simulink library "gsWave_cl"  (R2020a)
settings: Solver=VariableStepAuto  StartTime=0.0  StopTime=10.0  RelTol=1e-3
undefined symbols (not defined in the file): gndStn
libraries: eulAng2RotMat_ul x1, simulink x1, firstOrdTrnsThm_ul x1
settings Model: Creator=M.Cobb  LastModifiedBy=adabney
settings DataIOCC: ReturnWorkspaceOutputs=off
settings DebuggingCC: ArithmeticOperatorsInVariantConditions=warning
settings SFSimCC: CustomCodeUndefinedFunction=UseInterfaceOnly

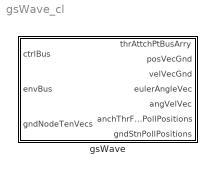
== system gsWave_cl ==
  gsWave : Subsystem  mask{gs=0}
      mask prompts: gs "Ground station object"

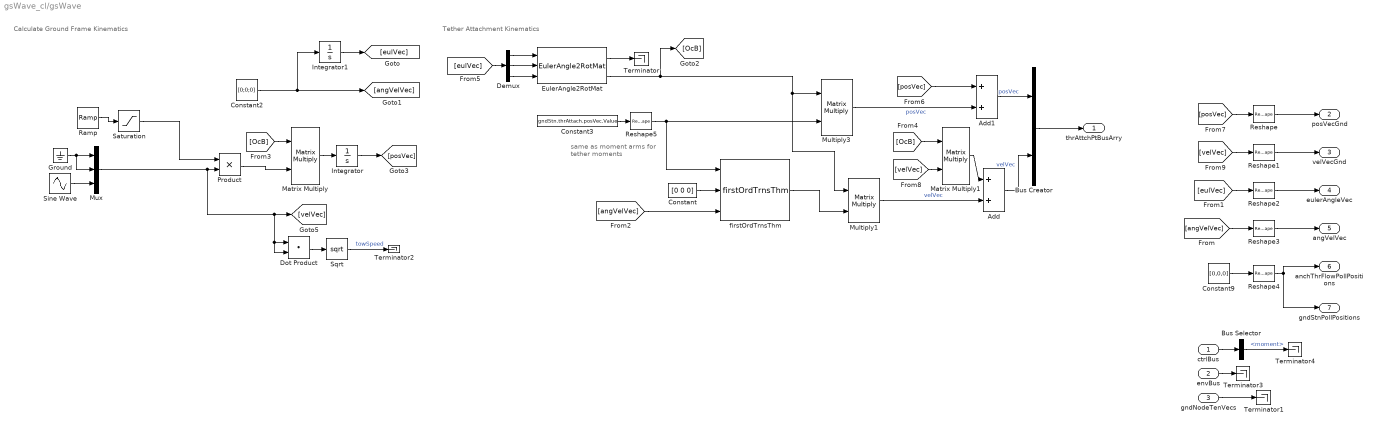
== system gsWave_cl/gsWave ==
  note: Tether Attachment Kinematics
  note: Calculate Ground Frame Kinematics
  note: same as moment arms
      | for tether moments
  ctrlBus : Inport  OutDataTypeStr=Bus: gndStnCtrlBus
  envBus : Inport  Port=2  OutDataTypeStr=Bus: envBus
  gndNodeTenVecs : Inport  Port=3
  Add : Sum
  Add1 : Sum
  Bus Creator : BusCreator  Inputs=2  OutDataTypeStr=Bus: thrAttachPtKinematicsBus  NonVirtualBus=on
  Bus Selector : BusSelector  OutputSignals=moment
  Constant : Constant  Value=[0 0 0]
  Constant2 : Constant  Value=[0;0;0]
  Constant3 : Constant  Value=gndStn.thrAttach.posVec.Value
  Constant9 : Constant  Value=[0,0,0]
  Demux : Demux  Outputs=3
  Dot Product : DotProduct  InputSameDT=on  OutDataTypeStr=Inherit: Inherit via internal rule
  EulerAngle2RotMat : eulAng2RotMat_ul/EulerAngle2RotMat  SystemSampleTime=-1  Latency=0  AutoFrameSizeCalculation=off
  Ground : Ground
  Integrator : Integrator  InitialCondition=gndStn.initPosVecGnd.Value
  Integrator1 : Integrator  InitialCondition=gndStn.initEulAng.Value
  Matrix Multiply : Product  Multiplication=Matrix(*)
  Matrix Multiply1 : Product  Multiplication=Matrix(*)
  Multiply1 : Product  Multiplication=Matrix(*)
  Multiply3 : Product  Multiplication=Matrix(*)
  Mux : Mux  Inputs=3
  Product : Product
  Ramp : simulink/Sources/Ramp  slope=0.05  start=0  InitialOutput=0
  Reshape{,1..5} (6 alike) : Reshape  OutputDimensionality=Column vector (2-D)
  Saturation : Saturate  UpperLimit=1  LowerLimit=0
  Sine Wave : Sin  Amplitude=gndStn.waveAmplitude.Value*2*pi/gndStn.wavePeriod.Value  Frequency=2*pi/gndStn.wavePeriod.Value  SampleTime=0
  Sqrt : Sqrt  SaturateOnIntegerOverflow=on
  Terminator{,1..4} (5 alike) : Terminator
  firstOrdTrnsThm : firstOrdTrnsThm_ul/firstOrdTrnsThm  SystemSampleTime=-1  Latency=0  AutoFrameSizeCalculation=off
  thrAttchPtBusArry : Outport  VectorParamsAs1DForOutWhenUnconnected=off
  posVecGnd : Outport  Port=2  VectorParamsAs1DForOutWhenUnconnected=off
  velVecGnd : Outport  Port=3  VectorParamsAs1DForOutWhenUnconnected=off
  eulerAngleVec : Outport  Port=4  VectorParamsAs1DForOutWhenUnconnected=off
  angVelVec : Outport  Port=5  VectorParamsAs1DForOutWhenUnconnected=off
  anchThrFlowPollPositions : Outport  Port=6  VectorParamsAs1DForOutWhenUnconnected=off
  gndStnPollPositions : Outport  Port=7  VectorParamsAs1DForOutWhenUnconnected=off
  wires:
  ctrlBus/1 -> Bus Selector/1
  envBus/1 -> Terminator3/1
  gndNodeTenVecs/1 -> Terminator1/1
  Reshape/1 -> posVecGnd/1
  Reshape1/1 -> velVecGnd/1
  Reshape2/1 -> eulerAngleVec/1
  Reshape3/1 -> angVelVec/1
  [angVelVec] -> Reshape3/1
  Bus Selector/1 -> Terminator4/1  "<moment>"
  Reshape4/1 -> anchThrFlowPollPositions/1, gndStnPollPositions/1
  Constant9/1 -> Reshape4/1
  [posVec] -> Reshape/1
  [velVec] -> Reshape1/1
  Mux/1 -> Product/2, Dot Product/2, Dot Product/1, [velVec]
  [eulVec] -> Reshape2/1
  EulerAngle2RotMat/1 -> Terminator/1
  Integrator1/1 -> [eulVec]
  Demux/3 -> EulerAngle2RotMat/3
  Demux/2 -> EulerAngle2RotMat/2
  Demux/1 -> EulerAngle2RotMat/1
  Add1/1 -> Bus Creator/1  "posVec"
  Constant/1 -> firstOrdTrnsThm/2
  Constant3/1 -> Reshape5/1
  firstOrdTrnsThm/1 -> Multiply1/2
  Reshape5/1 -> firstOrdTrnsThm/1, Multiply3/2
  Add/1 -> Bus Creator/2  "velVec"
  EulerAngle2RotMat/2 -> [OcB], Multiply1/1, Multiply3/1
  [velVec] -> Matrix Multiply1/2
  [posVec] -> Add1/1
  Multiply3/1 -> Add1/2  "posVec"
  Multiply1/1 -> Add/2  "velVec"
  Bus Creator/1 -> thrAttchPtBusArry/1
  [angVelVec] -> firstOrdTrnsThm/3
  [OcB] -> Matrix Multiply/1
  Matrix Multiply/1 -> Integrator/1
  Integrator/1 -> [posVec]
  Constant2/1 -> Integrator1/1, [angVelVec]
  [OcB] -> Matrix Multiply1/1
  [eulVec] -> Demux/1
  Matrix Multiply1/1 -> Add/1
  Dot Product/1 -> Sqrt/1
  Sqrt/1 -> Terminator2/1  "towSpeed"
  Ground/1 -> Mux/2, Mux/1
  Sine Wave/1 -> Mux/3
  Ramp/1 -> Saturation/1
  Saturation/1 -> Product/1
  Product/1 -> Matrix Multiply/2
